simulink model "Final_Completed_Assignment_Model_Zeeshan_Jamil"  (R2024a)
settings: Solver=ode4  StartTime=0.0  StopTime=10  FixedStep=0.01  RelTol=1e-3
settings Model: Creator=DELL  LastModifiedBy=DELL

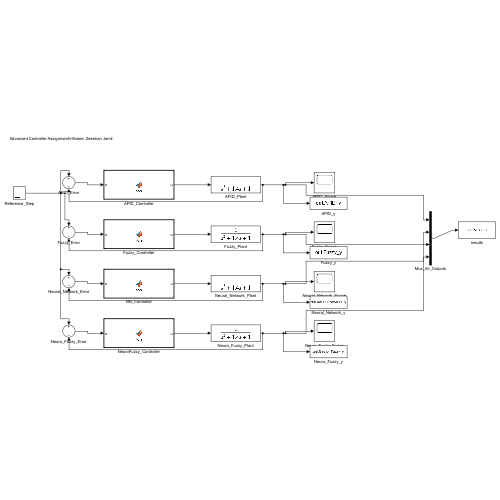
[thumbnail: Simulink's stored preview of the top-level diagram]
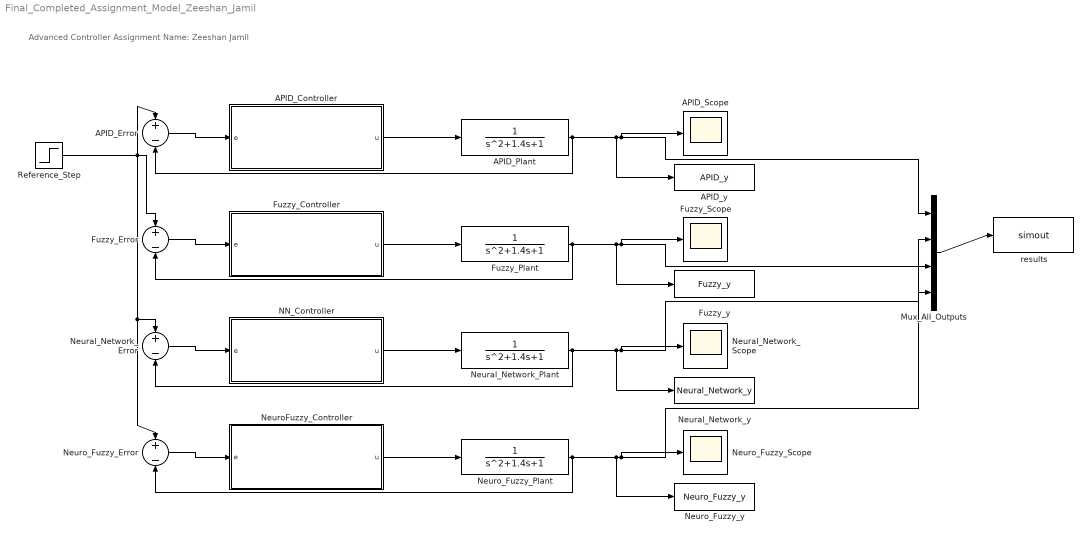
== system Final_Completed_Assignment_Model_Zeeshan_Jamil ==
  note: Advanced Controller Assignment\nName: Zeeshan Jamil
  APID_Controller : MATLAB Function  TreatAsAtomicUnit=on
  APID_Error : Sum  Inputs=+-
  APID_Plant : TransferFcn  Denominator=[1 1.4 1]
  APID_Scope : Scope
  APID_y : ToWorkspace  VariableName=APID_y  SaveFormat=Structure With Time  SampleTime=-1
  Fuzzy_Controller : MATLAB Function  TreatAsAtomicUnit=on
  Fuzzy_Error : Sum  Inputs=+-
  Fuzzy_Plant : TransferFcn  Denominator=[1 1.4 1]
  Fuzzy_Scope : Scope
  Fuzzy_y : ToWorkspace  VariableName=Fuzzy_y  SaveFormat=Structure With Time  SampleTime=-1
  Mux_All_Outputs : Mux
  NN_Controller : MATLAB Function  TreatAsAtomicUnit=on
  Neural_Network_Error : Sum  Inputs=+-
  Neural_Network_Plant : TransferFcn  Denominator=[1 1.4 1]
  Neural_Network_Scope : Scope
  Neural_Network_y : ToWorkspace  VariableName=Neural_Network_y  SaveFormat=Structure With Time  SampleTime=-1
  NeuroFuzzy_Controller : MATLAB Function  TreatAsAtomicUnit=on
  Neuro_Fuzzy_Error : Sum  Inputs=+-
  Neuro_Fuzzy_Plant : TransferFcn  Denominator=[1 1.4 1]
  Neuro_Fuzzy_Scope : Scope
  Neuro_Fuzzy_y : ToWorkspace  VariableName=Neuro_Fuzzy_y  SaveFormat=Structure With Time  SampleTime=-1
  Reference_Step : Step  Time=0  SampleTime=0
  results : ToWorkspace  VariableName=simout  SaveFormat=Structure With Time  SampleTime=-1
  wires:
  Mux_All_Outputs/1 -> results/1
  Reference_Step/1 -> Neural_Network_Error/1, Neuro_Fuzzy_Error/1, APID_Error/1, Fuzzy_Error/1
  APID_Error/1 -> APID_Controller/1(e)
  APID_Controller/1(u) -> APID_Plant/1
  APID_Plant/1 -> APID_Scope/1, Mux_All_Outputs/1, APID_y/1, APID_Error/2
  Fuzzy_Error/1 -> Fuzzy_Controller/1(e)
  Fuzzy_Controller/1(u) -> Fuzzy_Plant/1
  Fuzzy_Plant/1 -> Fuzzy_Scope/1, Mux_All_Outputs/2, Fuzzy_y/1, Fuzzy_Error/2
  Neural_Network_Error/1 -> NN_Controller/1(e)
  NN_Controller/1(u) -> Neural_Network_Plant/1
  Neural_Network_Plant/1 -> Neural_Network_Scope/1, Mux_All_Outputs/3, Neural_Network_y/1, Neural_Network_Error/2
  Neuro_Fuzzy_Error/1 -> NeuroFuzzy_Controller/1(e)
  NeuroFuzzy_Controller/1(u) -> Neuro_Fuzzy_Plant/1
  Neuro_Fuzzy_Plant/1 -> Neuro_Fuzzy_Scope/1, Mux_All_Outputs/4, Neuro_Fuzzy_y/1, Neuro_Fuzzy_Error/2

== matlab function Final_Completed_Assignment_Model_Zeeshan_Jamil/APID_Controller ==
  settings: updateMethod=DISCRETE
  data: e input; u output
function u = fcn(e)                                                  
                                                                    % Adaptive PID Controller with Higher Gain                           
                                                                    % Single Input : e                                                   
                                                                    % Single Output: u                                                   
                                                                    %                                                                    
                                                                    % This version uses significantly higher gains so the output sinusoid
                                                                    % closely matches the reference amplitude and phase.                 
                                                                    persistent Kp Ki Kd                                                  
                                                                    persistent e_prev integral_e d_filt u_prev                           
                                                                    persistent Ts                                                        
                                                                    if isempty(Kp)                                                       
                                                                        Kp = 20.0;                                                       
                                                                        Ki = 1.0;                                                        
                                                                        Kd = 0.2;                                                        
                                                                        e_prev     = 0;                                                  
                                                                        integral_e = 0;                                                  
                                                                        d_filt     = 0;                                                  
                                                                        u_prev     = 0;                                                  
                                                                        Ts = 0.01;                                                       
                                                                    end                                                                  
                                                                    eta_p = 1e-6;                                                        
                                                                    eta_i = 5e-8;                                                        
                                                                    eta_d = 5e-8;                                                        
                                                                    E_MAX = 1.5;                                                         
                                                                    e = min(max(e, -E_MAX), E_MAX);                                      
                                                                    integral_e = integral_e + e * Ts;                                    
                                                                    integral_e = min(max(integral_e, -10), 10);                          
                                                                    raw_d = (e - e_prev) / Ts;                                           
                                                                    alpha_d = 0.98;                                                      
                                                                    d_filt = alpha_d * d_filt + (1 - alpha_d) * raw_d;                   
                                                                    Kp = Kp + eta_p * e^2;                                               
                                                                    Ki = Ki + eta_i * e * integral_e;                                    
                                                                    Kd = Kd + eta_d * e * d_filt;                                        
                                                                    Kp = min(max(Kp, 0), 50);                                            
                                                                    Ki = min(max(Ki, 0), 5);                                             
                                                                    Kd = min(max(Kd, 0), 2);                                             
                                                                    u_raw = Kp * e + Ki * integral_e + Kd * d_filt;                      
                                                                    U_MAX = 1.05;                                                        
                                                                    scale = 0.5;                                                         
                                                                    u_sat = U_MAX * tanh(u_raw / scale);                                 
                                                                    beta = 0.85;                                                         
                                                                    u = beta * u_prev + (1 - beta) * u_sat;                              
                                                                    u_prev = u;                                                          
                                                                    e_prev = e;                                                          
                                                                    end

== matlab function Final_Completed_Assignment_Model_Zeeshan_Jamil/NN_Controller ==
  settings: updateMethod=DISCRETE
  data: e input; u output
function u = fcn(e)
% Online neural controller: 2-input, 5-hidden-node MLP
persistent ep Ts W1 b1 W2 b2 eta
if isempty(W1)
 Ts=0.01; eta=0.01; ep=0;
 W1=[0.5 -0.3; -0.4 0.2; 0.1 0.5; -0.2 -0.4; 0.3 0.1]; b1=zeros(5,1); W2=[1 -1 0.5 -0.5 0.2]; b2=0;
end
x=[e; (e-ep)/Ts/10]; h=tanh(W1*x+b1); u=W2*h+b2;
% Supervised target approximates a stabilizing PD action
target=7*e+0.25*(e-ep)/Ts; err=target-u;
W2=W2+eta*err*h'; b2=b2+eta*err;
g=(1-h.^2).*(W2'*err); W1=W1+eta*g*x'; b1=b1+eta*g;
u=min(max(u,-10),10); ep=e;
end

== matlab function Final_Completed_Assignment_Model_Zeeshan_Jamil/NeuroFuzzy_Controller ==
  settings: updateMethod=DISCRETE
  data: e input; u output
function u = fcn(e)
% First-order Sugeno neuro-fuzzy controller with normalized firing strengths
persistent ep Ts p eta
if isempty(p), Ts=0.01; ep=0; eta=0.02; p=[-6 0 6; -3 0 3; -1 0 1]; end
de=(e-ep)/Ts/10; muE=tri3(max(min(e,1),-1)); muD=tri3(max(min(de,1),-1));
num=0; den=0; phi=zeros(3,3);
for i=1:3
 for j=1:3
  phi(i,j)=muE(i)*muD(j); num=num+phi(i,j)*p(i,j); den=den+phi(i,j);
 end
end
u=num/(den+eps);
% Consequent adaptation drives output in error-reducing direction
p = p + eta*e*phi/(den+eps);
u=min(max(u,-10),10); ep=e;
end
function m=tri3(x)
m=[max(0,min(1,-x)), max(0,1-abs(x)), max(0,min(1,x))];
end

== matlab function Final_Completed_Assignment_Model_Zeeshan_Jamil/Fuzzy_Controller ==
  settings: updateMethod=DISCRETE
  data: e input; u output
function u = fcn(e)
% Mamdani-like fuzzy PD using triangular membership rules
persistent ep Ts
if isempty(ep), ep=0; Ts=0.01; end
de = (e-ep)/Ts;
centers = [-1 0 1];
muE = tri3(max(min(e,1),-1)); muD = tri3(max(min(de/5,1),-1));
rule = [-1 -0.7 0; -0.7 0 0.7; 0 0.7 1];
num=0; den=0;
for i=1:3
  for j=1:3
    w = muE(i)*muD(j); num = num + w*rule(i,j); den = den + w;
  end
end
u = 7*num/(den+eps);
ep=e;
end
function m=tri3(x)
m = [max(0,min(1,-x)), max(0,1-abs(x)), max(0,min(1,x))];
end
